simulink model "ACC_FFNN_trainlm_10_10_10_10_Nor_Sat_Feb_15"  (R2021a)
settings: Solver=FixedStepAuto  StartTime=0.0  StopTime=T  RelTol=1e-3
InitFcn:
  | seed = randi(10000);
StartFcn:
  | seed = randi(10000);
undefined symbols (not defined in the file): amax_ego, amin_ego, t_gap, Ts, v0_ego, v0_lead, v_set, x0_ego, x0_lead, x_gain, x_offset, y_gain, y_offset
libraries: neural x46
(part 2 of 2)

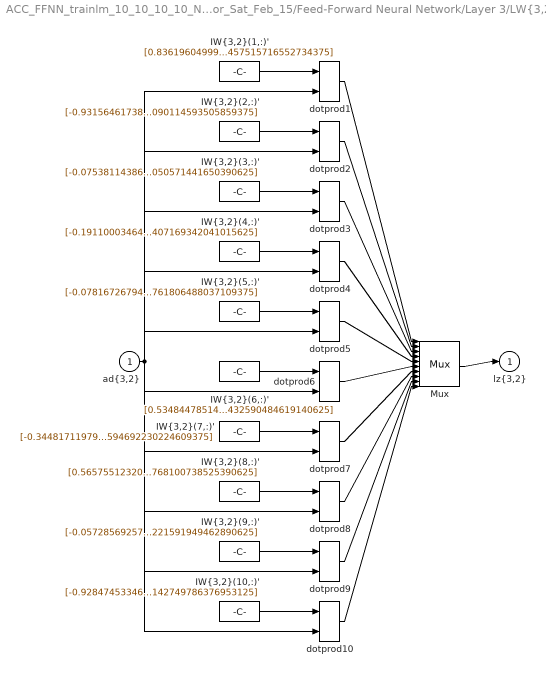
== system ACC_FFNN_trainlm_10_10_10_10_Nor_Sat_Feb_15/Feed-Forward Neural Network/Layer 3/LW{3,2} ==
  "ad{3,2}" : Inport  PortDimensions=10
      mask Display: e = 0.06;c1 = [120 230 180]/255;c2 = ([120 230 180]+0)/(256+128);c3 = ([120 230 180]+128)/(256+128);patch([0 1 1 0],[0 0 1 1],c1);patch([0 1 1 1-e 1-e 0+e],[0 0 1 1-e 0+e 0+e],c2);patch([0 0 1 1-e 0+e 0+e],[0 1 1 1-e 1-e 0+e],c3);plot([0 1 1 0 0],[0 0 1 1 0]);
  "IW{3,2}(1,:)'" : Constant  Value=[0.8361960499970726434781909119919873774051666259765625;-0.6482511686329381905835589350317604839801788330078125;-1.13250609637896371140186602133326232433319091796875;-0.422460691105411345613873663751292042434215545654296875;-0.08346649784732977639389872592801111750304698944091796875;0.217152453805795619956597874988801777362823486328125;-0.50238807137207874831119625014252960681915283203125;-0.1908400082847483414383304989314638078212738037109375;0.39331737625027740623551153476000763475894927978515625;-0.379503086542249457036035664714290760457515716552734375]
      mask Display: e = 0.06;c1 = [120 150 230]/255;c2 = ([120 150 230]+0)/383;c3 = ([120 150 230]+128)/383;patch([0 1 1 0],[0 0 1 1],c1);patch([0 1 1 1-e 1-e 0+e],[0 0 1 1-e 0+e 0+e],c2);patch([0 0 1 1-e 0+e 0+e],[0 1 1 1-e 1-e 0+e],c3);plot([0 1 1 0 0],[0 0 1 1 0]);disp('weights');
  "IW{3,2}(10,:)'" : Constant  Value=[-0.92847453346176411770329650607891380786895751953125;0.834848684098764781680301894084550440311431884765625;0.288885562862672973238886697799898684024810791015625;-0.0997246060682079882298012307728640735149383544921875;0.226921473625750547142843061010353267192840576171875;0.27863392208021675600093658431433141231536865234375;-0.872817258049788602392027314635924994945526123046875;-0.7222515943416893957618185595492832362651824951171875;0.040104934780773593416824951418675482273101806640625;-0.2815435791962788147912988279131241142749786376953125]
      mask Display: e = 0.06;c1 = [120 150 230]/255;c2 = ([120 150 230]+0)/383;c3 = ([120 150 230]+128)/383;patch([0 1 1 0],[0 0 1 1],c1);patch([0 1 1 1-e 1-e 0+e],[0 0 1 1-e 0+e 0+e],c2);patch([0 0 1 1-e 0+e 0+e],[0 1 1 1-e 1-e 0+e],c3);plot([0 1 1 0 0],[0 0 1 1 0]);disp('weights');
  "IW{3,2}(2,:)'" : Constant  Value=[-0.93156461738395235361309687505126930773258209228515625;0.443516066782204898544250681879930198192596435546875;0.81548873981788994047548158050631172955036163330078125;0.810982307606329388960375581518746912479400634765625;0.3253323371790364237909898292855359613895416259765625;-0.366009714119647167063220649652066640555858612060546875;0.494516689959643873653050150096532888710498809814453125;-0.1032541758670093567928915945230983197689056396484375;-0.80746129497860241741591380559839308261871337890625;-0.67959169216580261885241043273708783090114593505859375]
      mask Display: e = 0.06;c1 = [120 150 230]/255;c2 = ([120 150 230]+0)/383;c3 = ([120 150 230]+128)/383;patch([0 1 1 0],[0 0 1 1],c1);patch([0 1 1 1-e 1-e 0+e],[0 0 1 1-e 0+e 0+e],c2);patch([0 0 1 1-e 0+e 0+e],[0 1 1 1-e 1-e 0+e],c3);plot([0 1 1 0 0],[0 0 1 1 0]);disp('weights');
  "IW{3,2}(3,:)'" : Constant  Value=[-0.07538114386957632528929451609656098298728466033935546875;-0.05302801406935930828012715210206806659698486328125;-1.666466424504951415741516029811464250087738037109375;-0.5494592643148232813388176509761251509189605712890625;0.53818542754949005857412203113199211657047271728515625;1.437012642607873313949085058993659913539886474609375;-1.32599230539876433709878256195224821567535400390625;-0.2683676463236575049364773803972639143466949462890625;0.05957884425177140119700425202609039843082427978515625;0.06288604269901033883005680991118424572050571441650390625]
      mask Display: e = 0.06;c1 = [120 150 230]/255;c2 = ([120 150 230]+0)/383;c3 = ([120 150 230]+128)/383;patch([0 1 1 0],[0 0 1 1],c1);patch([0 1 1 1-e 1-e 0+e],[0 0 1 1-e 0+e 0+e],c2);patch([0 0 1 1-e 0+e 0+e],[0 1 1 1-e 1-e 0+e],c3);plot([0 1 1 0 0],[0 0 1 1 0]);disp('weights');
  "IW{3,2}(4,:)'" : Constant  Value=[-0.1911000346439272468135328608695999719202518463134765625;-0.6945575991235364288201026283786632120609283447265625;0.430956824004506688918780810126918368041515350341796875;1.3157701026058499227389120278530754148960113525390625;-0.299544251126169225329931578016839921474456787109375;-0.06099190108768766382940640369270113296806812286376953125;0.26342982208948029221318165582488290965557098388671875;0.5270092816976268412787476336234249174594879150390625;0.054098228565367452447265605997017701156437397003173828125;-0.37006111156151233476663264809758402407169342041015625]
      mask Display: e = 0.06;c1 = [120 150 230]/255;c2 = ([120 150 230]+0)/383;c3 = ([120 150 230]+128)/383;patch([0 1 1 0],[0 0 1 1],c1);patch([0 1 1 1-e 1-e 0+e],[0 0 1 1-e 0+e 0+e],c2);patch([0 0 1 1-e 0+e 0+e],[0 1 1 1-e 1-e 0+e],c3);plot([0 1 1 0 0],[0 0 1 1 0]);disp('weights');
  "IW{3,2}(5,:)'" : Constant  Value=[-0.0781672679420719607179535159957595169544219970703125;-0.3177507859017814073609997649327851831912994384765625;-0.81777307262693010869725185330025851726531982421875;-0.582130155147954297945034340955317020416259765625;0.32401919671826906466094442293979227542877197265625;-0.363851849037881702741970002534799277782440185546875;0.0449906115542042517319032413070090115070343017578125;0.25579275922833755174679026822559535503387451171875;0.722279622786664798894662453676573932170867919921875;-0.9110918154435230231769082820392213761806488037109375]
      mask Display: e = 0.06;c1 = [120 150 230]/255;c2 = ([120 150 230]+0)/383;c3 = ([120 150 230]+128)/383;patch([0 1 1 0],[0 0 1 1],c1);patch([0 1 1 1-e 1-e 0+e],[0 0 1 1-e 0+e 0+e],c2);patch([0 0 1 1-e 0+e 0+e],[0 1 1 1-e 1-e 0+e],c3);plot([0 1 1 0 0],[0 0 1 1 0]);disp('weights');
  "IW{3,2}(6,:)'" : Constant  Value=[0.5348447851462225788310433927108533680438995361328125;0.2147784275366948492091978550888597965240478515625;0.15674699215131615570584244778729043900966644287109375;0.41865402547300722968515174216008745133876800537109375;-0.1720782038018791870737089766407734714448451995849609375;-0.78317252089697275696522638099850155413150787353515625;1.032454614753462340814849085290916264057159423828125;0.54396077110849017088867185520939528942108154296875;-0.030293332895796165615820427774451673030853271484375;0.50269902741955763136871837559738196432590484619140625]
      mask Display: e = 0.06;c1 = [120 150 230]/255;c2 = ([120 150 230]+0)/383;c3 = ([120 150 230]+128)/383;patch([0 1 1 0],[0 0 1 1],c1);patch([0 1 1 1-e 1-e 0+e],[0 0 1 1-e 0+e 0+e],c2);patch([0 0 1 1-e 0+e 0+e],[0 1 1 1-e 1-e 0+e],c3);plot([0 1 1 0 0],[0 0 1 1 0]);disp('weights');
  "IW{3,2}(7,:)'" : Constant  Value=[-0.34481711979075824192619847963214851915836334228515625;-0.616509489076404459950708769611082971096038818359375;0.34156660969493335411328871487057767808437347412109375;-0.52747681944062130288131129418616183102130889892578125;0.6838583053826179369849569411599077284336090087890625;0.879658940689841184479291769093833863735198974609375;-0.56264673520073227308557761716656386852264404296875;0.8657071405576390876746017966070212423801422119140625;-0.213087277569467214988208070280961692333221435546875;-0.5144292843580762220057067679590545594692230224609375]
      mask Display: e = 0.06;c1 = [120 150 230]/255;c2 = ([120 150 230]+0)/383;c3 = ([120 150 230]+128)/383;patch([0 1 1 0],[0 0 1 1],c1);patch([0 1 1 1-e 1-e 0+e],[0 0 1 1-e 0+e 0+e],c2);patch([0 0 1 1-e 0+e 0+e],[0 1 1 1-e 1-e 0+e],c3);plot([0 1 1 0 0],[0 0 1 1 0]);disp('weights');
  "IW{3,2}(8,:)'" : Constant  Value=[0.565755123208306454074545399635098874568939208984375;0.476853679953883169417849785531871020793914794921875;0.104547087801231286530168063109158538281917572021484375;-0.75662029737058966727403230834170244634151458740234375;0.6658336381504315060197995990165509283542633056640625;0.29110374994504706336329036275856196880340576171875;-0.7884034534995436604987162354518659412860870361328125;0.945481708006027599111575909773819148540496826171875;0.342862279348052023664195075980387628078460693359375;-0.125218019142410208477400601623230613768100738525390625]
      mask Display: e = 0.06;c1 = [120 150 230]/255;c2 = ([120 150 230]+0)/383;c3 = ([120 150 230]+128)/383;patch([0 1 1 0],[0 0 1 1],c1);patch([0 1 1 1-e 1-e 0+e],[0 0 1 1-e 0+e 0+e],c2);patch([0 0 1 1-e 0+e 0+e],[0 1 1 1-e 1-e 0+e],c3);plot([0 1 1 0 0],[0 0 1 1 0]);disp('weights');
  "IW{3,2}(9,:)'" : Constant  Value=[-0.057285692578776803429718711413443088531494140625;-0.514300803363661795941652599140070378780364990234375;-0.1485423162576242628318823335575871169567108154296875;0.21460788137126929342457515303976833820343017578125;-0.4871180155417054180588820599950850009918212890625;-0.0410735501022243543189915726543404161930084228515625;-0.7806050709536116460895982527290470898151397705078125;-0.6159433011444501726572298139217309653759002685546875;0.4825158869084129609206001987331546843051910400390625;0.3755921702402142958732156330370344221591949462890625]
      mask Display: e = 0.06;c1 = [120 150 230]/255;c2 = ([120 150 230]+0)/383;c3 = ([120 150 230]+128)/383;patch([0 1 1 0],[0 0 1 1],c1);patch([0 1 1 1-e 1-e 0+e],[0 0 1 1-e 0+e 0+e],c2);patch([0 0 1 1-e 0+e 0+e],[0 1 1 1-e 1-e 0+e],c3);plot([0 1 1 0 0],[0 0 1 1 0]);disp('weights');
  Mux : Mux  Inputs=10
      mask Display: e = 0.06;c1 = [120 150 230]/255;c2 = ([120 150 230]+0)/383;c3 = ([120 150 230]+128)/383;patch([0 1 1 0],[0 0 1 1],c1);patch([0 1 1 1-e 1-e 0+e],[0 0 1 1-e 0+e 0+e],c2);patch([0 0 1 1-e 0+e 0+e],[0 1 1 1-e 1-e 0+e],c3);plot([0 1 1 0 0],[0 0 1 1 0]);disp('Mux');
  dotprod{1..10} (10 alike) : neural/Weight Functions/dotprod
  "lz{3,2}" : Outport
      mask Display: e = 0.06;c1 = [120 230 180]/255;c2 = ([120 230 180]+0)/(256+128);c3 = ([120 230 180]+128)/(256+128);patch([0 1 1 0],[0 0 1 1],c1);patch([0 1 1 1-e 1-e 0+e],[0 0 1 1-e 0+e 0+e],c2);patch([0 0 1 1-e 0+e 0+e],[0 1 1 1-e 1-e 0+e],c3);plot([0 1 1 0 0],[0 0 1 1 0]);
  wires:
  "IW{3,2}(1,:)'"/1 -> dotprod1/1
  "ad{3,2}"/1 -> dotprod1/2, dotprod2/2, dotprod3/2, dotprod4/2, dotprod5/2, dotprod6/2, dotprod7/2, dotprod8/2, dotprod9/2, dotprod10/2
  dotprod1/1 -> Mux/1
  "IW{3,2}(2,:)'"/1 -> dotprod2/1
  dotprod2/1 -> Mux/2
  "IW{3,2}(3,:)'"/1 -> dotprod3/1
  dotprod3/1 -> Mux/3
  "IW{3,2}(4,:)'"/1 -> dotprod4/1
  dotprod4/1 -> Mux/4
  "IW{3,2}(5,:)'"/1 -> dotprod5/1
  dotprod5/1 -> Mux/5
  "IW{3,2}(6,:)'"/1 -> dotprod6/1
  dotprod6/1 -> Mux/6
  "IW{3,2}(7,:)'"/1 -> dotprod7/1
  dotprod7/1 -> Mux/7
  "IW{3,2}(8,:)'"/1 -> dotprod8/1
  dotprod8/1 -> Mux/8
  "IW{3,2}(9,:)'"/1 -> dotprod9/1
  dotprod9/1 -> Mux/9
  "IW{3,2}(10,:)'"/1 -> dotprod10/1
  dotprod10/1 -> Mux/10
  Mux/1 -> "lz{3,2}"/1

== system ACC_FFNN_trainlm_10_10_10_10_Nor_Sat_Feb_15/Feed-Forward Neural Network/Layer 4/Delays 1 ==
  "p{4}" : Inport  PortDimensions=10
      mask Display: e = 0.06;c1 = [120 230 180]/255;c2 = ([120 230 180]+0)/(256+128);c3 = ([120 230 180]+128)/(256+128);patch([0 1 1 0],[0 0 1 1],c1);patch([0 1 1 1-e 1-e 0+e],[0 0 1 1-e 0+e 0+e],c2);patch([0 0 1 1-e 0+e 0+e],[0 1 1 1-e 1-e 0+e],c3);plot([0 1 1 0 0],[0 0 1 1 0]);
  mux : Mux  Inputs=1
      mask Display: e = 0.06;c1 = [120 150 230]/255;c2 = ([120 150 230]+0)/383;c3 = ([120 150 230]+128)/383;patch([0 1 1 0],[0 0 1 1],c1);patch([0 1 1 1-e 1-e 0+e],[0 0 1 1-e 0+e 0+e],c2);patch([0 0 1 1-e 0+e 0+e],[0 1 1 1-e 1-e 0+e],c3);plot([0 1 1 0 0],[0 0 1 1 0]);disp('Mux')
  "pd{4,3}" : Outport
      mask Display: e = 0.06;c1 = [120 230 180]/255;c2 = ([120 230 180]+0)/(256+128);c3 = ([120 230 180]+128)/(256+128);patch([0 1 1 0],[0 0 1 1],c1);patch([0 1 1 1-e 1-e 0+e],[0 0 1 1-e 0+e 0+e],c2);patch([0 0 1 1-e 0+e 0+e],[0 1 1 1-e 1-e 0+e],c3);plot([0 1 1 0 0],[0 0 1 1 0]);
  wires:
  "p{4}"/1 -> mux/1
  mux/1 -> "pd{4,3}"/1

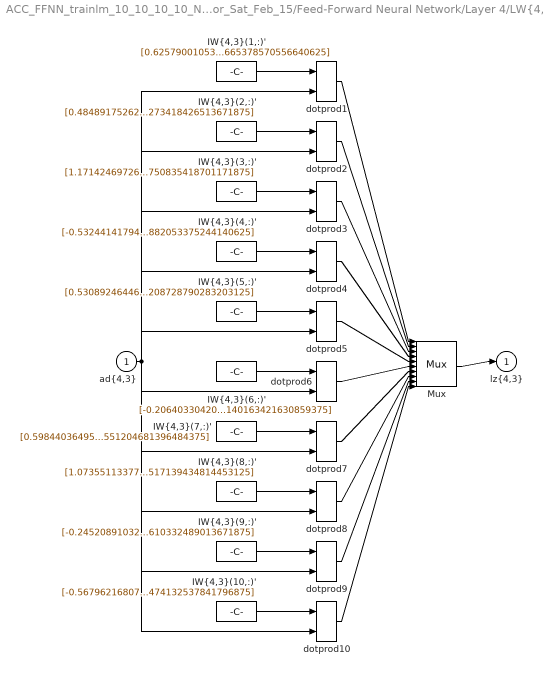
== system ACC_FFNN_trainlm_10_10_10_10_Nor_Sat_Feb_15/Feed-Forward Neural Network/Layer 4/LW{4,3} ==
  "ad{4,3}" : Inport  PortDimensions=10
      mask Display: e = 0.06;c1 = [120 230 180]/255;c2 = ([120 230 180]+0)/(256+128);c3 = ([120 230 180]+128)/(256+128);patch([0 1 1 0],[0 0 1 1],c1);patch([0 1 1 1-e 1-e 0+e],[0 0 1 1-e 0+e 0+e],c2);patch([0 0 1 1-e 0+e 0+e],[0 1 1 1-e 1-e 0+e],c3);plot([0 1 1 0 0],[0 0 1 1 0]);
  "IW{4,3}(1,:)'" : Constant  Value=[0.6257900105325717721171940866042859852313995361328125;0.58766425315506498616713315641391091048717498779296875;-0.000500402411035343074909020888441091301501728594303131103515625;0.0445499800293158443320606920678983442485332489013671875;0.7014253485780148622552587767131626605987548828125;0.23846823339999201341043999491375871002674102783203125;0.47728058399080364182509583770297467708587646484375;0.5380581706717924017624454791075550019741058349609375;0.1045826830775500315695580866304226219654083251953125;-0.7069701787702202810947937905439175665378570556640625]
      mask Display: e = 0.06;c1 = [120 150 230]/255;c2 = ([120 150 230]+0)/383;c3 = ([120 150 230]+128)/383;patch([0 1 1 0],[0 0 1 1],c1);patch([0 1 1 1-e 1-e 0+e],[0 0 1 1-e 0+e 0+e],c2);patch([0 0 1 1-e 0+e 0+e],[0 1 1 1-e 1-e 0+e],c3);plot([0 1 1 0 0],[0 0 1 1 0]);disp('weights');
  "IW{4,3}(10,:)'" : Constant  Value=[-0.56796216807721133790209933067671954631805419921875;0.9797443072630078741980241829878650605678558349609375;-0.3629515092020156874497160970349796116352081298828125;-0.890051706187623636878925026394426822662353515625;0.7308771820260491214327203124412335455417633056640625;0.6903563701080732695203323601162992417812347412109375;0.964606445767212772324228353681974112987518310546875;-0.581189831958130564970588238793425261974334716796875;-0.5890116581846402965538800344802439212799072265625;-0.10963366940791541281896570581011474132537841796875]
      mask Display: e = 0.06;c1 = [120 150 230]/255;c2 = ([120 150 230]+0)/383;c3 = ([120 150 230]+128)/383;patch([0 1 1 0],[0 0 1 1],c1);patch([0 1 1 1-e 1-e 0+e],[0 0 1 1-e 0+e 0+e],c2);patch([0 0 1 1-e 0+e 0+e],[0 1 1 1-e 1-e 0+e],c3);plot([0 1 1 0 0],[0 0 1 1 0]);disp('weights');
  "IW{4,3}(2,:)'" : Constant  Value=[0.484891752629080186043353251079679466784000396728515625;0.50896011869223178880616842434392310678958892822265625;1.521302019557283724537910529761575162410736083984375;-0.7951717772056221544829668346210382878780364990234375;0.1211190547097695802136740894638933241367340087890625;0.964077572357958434423608196084387600421905517578125;0.1726188334970764903797402212148881517350673675537109375;0.1942421228665956733916431176112382672727108001708984375;0.25976677012884241690926501178182661533355712890625;-0.621855651054772362584799338947050273418426513671875]
      mask Display: e = 0.06;c1 = [120 150 230]/255;c2 = ([120 150 230]+0)/383;c3 = ([120 150 230]+128)/383;patch([0 1 1 0],[0 0 1 1],c1);patch([0 1 1 1-e 1-e 0+e],[0 0 1 1-e 0+e 0+e],c2);patch([0 0 1 1-e 0+e 0+e],[0 1 1 1-e 1-e 0+e],c3);plot([0 1 1 0 0],[0 0 1 1 0]);disp('weights');
  "IW{4,3}(3,:)'" : Constant  Value=[1.171424697267141379342092477600090205669403076171875;-0.56737731599117946501564802019856870174407958984375;0.429402168276678708469518142010201700031757354736328125;-0.87361313832371145782218491149251349270343780517578125;0.8592177335133264204358738425071351230144500732421875;0.05907996221176241291583863812775234691798686981201171875;-0.50779337195259277581982360061374492943286895751953125;0.8510792221733556317531110835261642932891845703125;-0.9360179684748661799176261411048471927642822265625;-0.9146951781777132861606105507235042750835418701171875]
      mask Display: e = 0.06;c1 = [120 150 230]/255;c2 = ([120 150 230]+0)/383;c3 = ([120 150 230]+128)/383;patch([0 1 1 0],[0 0 1 1],c1);patch([0 1 1 1-e 1-e 0+e],[0 0 1 1-e 0+e 0+e],c2);patch([0 0 1 1-e 0+e 0+e],[0 1 1 1-e 1-e 0+e],c3);plot([0 1 1 0 0],[0 0 1 1 0]);disp('weights');
  "IW{4,3}(4,:)'" : Constant  Value=[-0.53244141794082633367679591174237430095672607421875;0.90327130074819284022424881186452694237232208251953125;-1.7648105127539583936169265143689699470996856689453125;-0.1826649796391853486365874914554296992719173431396484375;0.3933344011104551452007171974400989711284637451171875;-0.051931174047597207510396088991910801269114017486572265625;0.333398204397761743766892550411284901201725006103515625;0.167567088959138243975388604667386971414089202880859375;0.2294268382342810053131643144297413527965545654296875;0.270395833719764056013445951975882053375244140625]
      mask Display: e = 0.06;c1 = [120 150 230]/255;c2 = ([120 150 230]+0)/383;c3 = ([120 150 230]+128)/383;patch([0 1 1 0],[0 0 1 1],c1);patch([0 1 1 1-e 1-e 0+e],[0 0 1 1-e 0+e 0+e],c2);patch([0 0 1 1-e 0+e 0+e],[0 1 1 1-e 1-e 0+e],c3);plot([0 1 1 0 0],[0 0 1 1 0]);disp('weights');
  "IW{4,3}(5,:)'" : Constant  Value=[0.5308924644635764078515194341889582574367523193359375;-0.1406585780162202536924809237461886368691921234130859375;-0.6008378209976836803463129399460740387439727783203125;0.333907105617679444975465230527333915233612060546875;0.165581930351680117752266596653498709201812744140625;0.592735637027675732468878777581267058849334716796875;-0.8330343727947546739187600906006991863250732421875;-0.96603412332547744512112330994568765163421630859375;-0.2751770754538946928136056158109568059444427490234375;-0.4362662882391401542037101535242982208728790283203125]
      mask Display: e = 0.06;c1 = [120 150 230]/255;c2 = ([120 150 230]+0)/383;c3 = ([120 150 230]+128)/383;patch([0 1 1 0],[0 0 1 1],c1);patch([0 1 1 1-e 1-e 0+e],[0 0 1 1-e 0+e 0+e],c2);patch([0 0 1 1-e 0+e 0+e],[0 1 1 1-e 1-e 0+e],c3);plot([0 1 1 0 0],[0 0 1 1 0]);disp('weights');
  "IW{4,3}(6,:)'" : Constant  Value=[-0.2064033042026633679721925318517605774104595184326171875;0.6670546354820441337096781353466212749481201171875;-0.1860890741759412547740026866449625231325626373291015625;-0.009586178885343736577606676974028232507407665252685546875;0.6307944229548423376030541476211510598659515380859375;-0.54431412858791627940036050858907401561737060546875;0.25191957034316647678906520013697445392608642578125;-0.7582808578028836787865429869270883500576019287109375;-0.9009348419158775822523921306128613650798797607421875;0.07719335609068078696282100281678140163421630859375]
      mask Display: e = 0.06;c1 = [120 150 230]/255;c2 = ([120 150 230]+0)/383;c3 = ([120 150 230]+128)/383;patch([0 1 1 0],[0 0 1 1],c1);patch([0 1 1 1-e 1-e 0+e],[0 0 1 1-e 0+e 0+e],c2);patch([0 0 1 1-e 0+e 0+e],[0 1 1 1-e 1-e 0+e],c3);plot([0 1 1 0 0],[0 0 1 1 0]);disp('weights');
  "IW{4,3}(7,:)'" : Constant  Value=[0.598440364953251258128830158966593444347381591796875;0.27213804300464816687821212326525710523128509521484375;0.56630017205567517724063009154633618891239166259765625;-0.78261166391266867581322230762452818453311920166015625;0.7580278091943555285325828663189895451068878173828125;-0.0037654820676953902093553328001007685088552534580230712890625;0.321512605361214232058131301528192125260829925537109375;0.71278878636295772697195616274257190525531768798828125;-0.0208600216453564968333012075163424015045166015625;0.390326078888663996480090645491145551204681396484375]
      mask Display: e = 0.06;c1 = [120 150 230]/255;c2 = ([120 150 230]+0)/383;c3 = ([120 150 230]+128)/383;patch([0 1 1 0],[0 0 1 1],c1);patch([0 1 1 1-e 1-e 0+e],[0 0 1 1-e 0+e 0+e],c2);patch([0 0 1 1-e 0+e 0+e],[0 1 1 1-e 1-e 0+e],c3);plot([0 1 1 0 0],[0 0 1 1 0]);disp('weights');
  "IW{4,3}(8,:)'" : Constant  Value=[1.0735511337716570068323562736622989177703857421875;-1.09284610154307859630762322922237217426300048828125;1.6850028566631198856384799000807106494903564453125;-0.67244723172349962769800413298071362078189849853515625;0.9778232321591782127967462656670249998569488525390625;0.79495147985520520084179452169337309896945953369140625;0.459503710634442175120284446165896952152252197265625;-0.031406977575795025359184364788234233856201171875;-0.6149792078758504754176783535513095557689666748046875;-0.0017679730348210132007125139352865517139434814453125]
      mask Display: e = 0.06;c1 = [120 150 230]/255;c2 = ([120 150 230]+0)/383;c3 = ([120 150 230]+128)/383;patch([0 1 1 0],[0 0 1 1],c1);patch([0 1 1 1-e 1-e 0+e],[0 0 1 1-e 0+e 0+e],c2);patch([0 0 1 1-e 0+e 0+e],[0 1 1 1-e 1-e 0+e],c3);plot([0 1 1 0 0],[0 0 1 1 0]);disp('weights');
  "IW{4,3}(9,:)'" : Constant  Value=[-0.2452089103297943051273932724143378436565399169921875;0.72396095740414434516196706681512296199798583984375;0.579926059889061651375641304184682667255401611328125;-0.7047835560466226834108738330542109906673431396484375;-0.9989552492861104582289044628851115703582763671875;0.1493224382603752786735640256665647029876708984375;0.78150423265064450362160641816444694995880126953125;0.6897113491525264095116654061712324619293212890625;-0.753832504908109601871046834276057779788970947265625;0.071602111502226506445367704145610332489013671875]
      mask Display: e = 0.06;c1 = [120 150 230]/255;c2 = ([120 150 230]+0)/383;c3 = ([120 150 230]+128)/383;patch([0 1 1 0],[0 0 1 1],c1);patch([0 1 1 1-e 1-e 0+e],[0 0 1 1-e 0+e 0+e],c2);patch([0 0 1 1-e 0+e 0+e],[0 1 1 1-e 1-e 0+e],c3);plot([0 1 1 0 0],[0 0 1 1 0]);disp('weights');
  Mux : Mux  Inputs=10
      mask Display: e = 0.06;c1 = [120 150 230]/255;c2 = ([120 150 230]+0)/383;c3 = ([120 150 230]+128)/383;patch([0 1 1 0],[0 0 1 1],c1);patch([0 1 1 1-e 1-e 0+e],[0 0 1 1-e 0+e 0+e],c2);patch([0 0 1 1-e 0+e 0+e],[0 1 1 1-e 1-e 0+e],c3);plot([0 1 1 0 0],[0 0 1 1 0]);disp('Mux');
  dotprod{1..10} (10 alike) : neural/Weight Functions/dotprod
  "lz{4,3}" : Outport
      mask Display: e = 0.06;c1 = [120 230 180]/255;c2 = ([120 230 180]+0)/(256+128);c3 = ([120 230 180]+128)/(256+128);patch([0 1 1 0],[0 0 1 1],c1);patch([0 1 1 1-e 1-e 0+e],[0 0 1 1-e 0+e 0+e],c2);patch([0 0 1 1-e 0+e 0+e],[0 1 1 1-e 1-e 0+e],c3);plot([0 1 1 0 0],[0 0 1 1 0]);
  wires:
  "IW{4,3}(1,:)'"/1 -> dotprod1/1
  "ad{4,3}"/1 -> dotprod1/2, dotprod2/2, dotprod3/2, dotprod4/2, dotprod5/2, dotprod6/2, dotprod7/2, dotprod8/2, dotprod9/2, dotprod10/2
  dotprod1/1 -> Mux/1
  "IW{4,3}(2,:)'"/1 -> dotprod2/1
  dotprod2/1 -> Mux/2
  "IW{4,3}(3,:)'"/1 -> dotprod3/1
  dotprod3/1 -> Mux/3
  "IW{4,3}(4,:)'"/1 -> dotprod4/1
  dotprod4/1 -> Mux/4
  "IW{4,3}(5,:)'"/1 -> dotprod5/1
  dotprod5/1 -> Mux/5
  "IW{4,3}(6,:)'"/1 -> dotprod6/1
  dotprod6/1 -> Mux/6
  "IW{4,3}(7,:)'"/1 -> dotprod7/1
  dotprod7/1 -> Mux/7
  "IW{4,3}(8,:)'"/1 -> dotprod8/1
  dotprod8/1 -> Mux/8
  "IW{4,3}(9,:)'"/1 -> dotprod9/1
  dotprod9/1 -> Mux/9
  "IW{4,3}(10,:)'"/1 -> dotprod10/1
  dotprod10/1 -> Mux/10
  Mux/1 -> "lz{4,3}"/1

== system ACC_FFNN_trainlm_10_10_10_10_Nor_Sat_Feb_15/Feed-Forward Neural Network/Layer 5/Delays 1 ==
  "p{5}" : Inport  PortDimensions=10
      mask Display: e = 0.06;c1 = [120 230 180]/255;c2 = ([120 230 180]+0)/(256+128);c3 = ([120 230 180]+128)/(256+128);patch([0 1 1 0],[0 0 1 1],c1);patch([0 1 1 1-e 1-e 0+e],[0 0 1 1-e 0+e 0+e],c2);patch([0 0 1 1-e 0+e 0+e],[0 1 1 1-e 1-e 0+e],c3);plot([0 1 1 0 0],[0 0 1 1 0]);
  mux : Mux  Inputs=1
      mask Display: e = 0.06;c1 = [120 150 230]/255;c2 = ([120 150 230]+0)/383;c3 = ([120 150 230]+128)/383;patch([0 1 1 0],[0 0 1 1],c1);patch([0 1 1 1-e 1-e 0+e],[0 0 1 1-e 0+e 0+e],c2);patch([0 0 1 1-e 0+e 0+e],[0 1 1 1-e 1-e 0+e],c3);plot([0 1 1 0 0],[0 0 1 1 0]);disp('Mux')
  "pd{5,4}" : Outport
      mask Display: e = 0.06;c1 = [120 230 180]/255;c2 = ([120 230 180]+0)/(256+128);c3 = ([120 230 180]+128)/(256+128);patch([0 1 1 0],[0 0 1 1],c1);patch([0 1 1 1-e 1-e 0+e],[0 0 1 1-e 0+e 0+e],c2);patch([0 0 1 1-e 0+e 0+e],[0 1 1 1-e 1-e 0+e],c3);plot([0 1 1 0 0],[0 0 1 1 0]);
  wires:
  "p{5}"/1 -> mux/1
  mux/1 -> "pd{5,4}"/1

== system ACC_FFNN_trainlm_10_10_10_10_Nor_Sat_Feb_15/Feed-Forward Neural Network/Layer 5/LW{5,4} ==
  "ad{5,4}" : Inport  PortDimensions=10
      mask Display: e = 0.06;c1 = [120 230 180]/255;c2 = ([120 230 180]+0)/(256+128);c3 = ([120 230 180]+128)/(256+128);patch([0 1 1 0],[0 0 1 1],c1);patch([0 1 1 1-e 1-e 0+e],[0 0 1 1-e 0+e 0+e],c2);patch([0 0 1 1-e 0+e 0+e],[0 1 1 1-e 1-e 0+e],c3);plot([0 1 1 0 0],[0 0 1 1 0]);
  "IW{5,4}(1,:)'" : Constant  Value=[0.89867339799955081591775751803652383387088775634765625;-1.4213178096743046552319356123916804790496826171875;-1.4871247583480944332023909737472422420978546142578125;-1.7407901885078926884631300708861090242862701416015625;-0.65474733848296218230444765140418894588947296142578125;0.2419173037275011151070458481626701541244983673095703125;-0.46795818253836152234015344220097176730632781982421875;-2.269333800530727529576324741356074810028076171875;0.862402769216499276438980814418755471706390380859375;0.457323363356542333946208600536920130252838134765625]
      mask Display: e = 0.06;c1 = [120 150 230]/255;c2 = ([120 150 230]+0)/383;c3 = ([120 150 230]+128)/383;patch([0 1 1 0],[0 0 1 1],c1);patch([0 1 1 1-e 1-e 0+e],[0 0 1 1-e 0+e 0+e],c2);patch([0 0 1 1-e 0+e 0+e],[0 1 1 1-e 1-e 0+e],c3);plot([0 1 1 0 0],[0 0 1 1 0]);disp('weights');
  Mux : Mux  Inputs=1
      mask Display: e = 0.06;c1 = [120 150 230]/255;c2 = ([120 150 230]+0)/383;c3 = ([120 150 230]+128)/383;patch([0 1 1 0],[0 0 1 1],c1);patch([0 1 1 1-e 1-e 0+e],[0 0 1 1-e 0+e 0+e],c2);patch([0 0 1 1-e 0+e 0+e],[0 1 1 1-e 1-e 0+e],c3);plot([0 1 1 0 0],[0 0 1 1 0]);disp('Mux');
  dotprod1 : neural/Weight Functions/dotprod
  "lz{5,4}" : Outport
      mask Display: e = 0.06;c1 = [120 230 180]/255;c2 = ([120 230 180]+0)/(256+128);c3 = ([120 230 180]+128)/(256+128);patch([0 1 1 0],[0 0 1 1],c1);patch([0 1 1 1-e 1-e 0+e],[0 0 1 1-e 0+e 0+e],c2);patch([0 0 1 1-e 0+e 0+e],[0 1 1 1-e 1-e 0+e],c3);plot([0 1 1 0 0],[0 0 1 1 0]);
  wires:
  "IW{5,4}(1,:)'"/1 -> dotprod1/1
  "ad{5,4}"/1 -> dotprod1/2
  dotprod1/1 -> Mux/1
  Mux/1 -> "lz{5,4}"/1
